simulink model "logicandbit"  (R2024b)
settings: Solver=FixedStepAuto  StartTime=0.0  StopTime=10.0  FixedStep=0.1  RelTol=1e-3
libraries: simulink x3
settings Model: Creator=Minkyo  LastModifiedBy=Minkyo

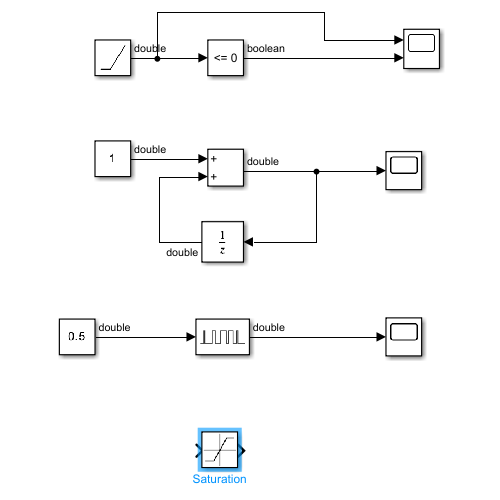
[thumbnail: Simulink's stored preview of the top-level diagram]
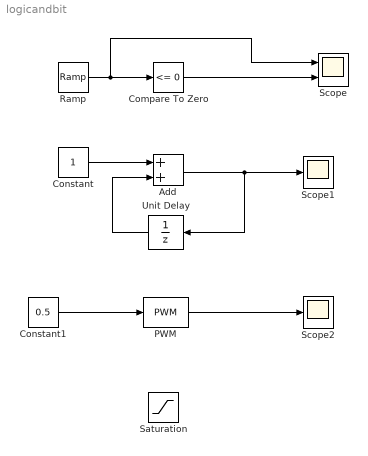
== system logicandbit ==
  Add : Sum
  Compare To Zero : simulink/Logic and Bit Operations/Compare To Zero  relop=<=  OutDataTypeStr=boolean
  Constant : Constant
  Constant1 : Constant  Value=0.5
  PWM : simulink/Discontinuities/PWM  DisableCoverage=on  Period=1  InitialDelay=0  DisallowZeroDutyCycle=off  RunAtFixedTimeIntervals=on  SampleTime=0.1
  Ramp : simulink/Sources/Ramp  slope=4  start=3  InitialOutput=0
  Saturation : Saturate
  Scope : Scope  NumInputPorts=2
  Scope1 : Scope
  Scope2 : Scope
  Unit Delay : UnitDelay  SampleTime=-1  HasFrameUpgradeWarning=on
  wires:
  Ramp/1 -> Scope/1, Compare To Zero/1
  Compare To Zero/1 -> Scope/2
  Constant/1 -> Add/1
  Add/1 -> Unit Delay/1, Scope1/1
  Unit Delay/1 -> Add/2
  Constant1/1 -> PWM/1
  PWM/1 -> Scope2/1
